simulink model "sine_test_sin_ideal"  (R2023b)
settings: Solver=FixedStepAuto  StartTime=0.0  StopTime=SimTime  FixedStep=samplingTime  RelTol=1e-3
values from neighbouring files (symbols this model uses):
  M = -max(y_norm)    [Fractional_contr.m]
  Omega = 2*pi*freq    (= 1.13097335529)    [Fractional_contr.m]
  Phi = freq*2*pi*( (27918-28129)*samplingTime )    (= -2.38635377967)    [Fractional_contr.m]
settings Model: Creator=tudor  LastModifiedBy=tudor

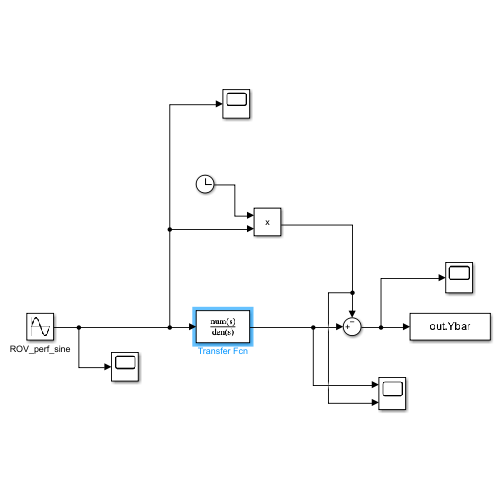
[thumbnail: Simulink's stored preview of the top-level diagram]
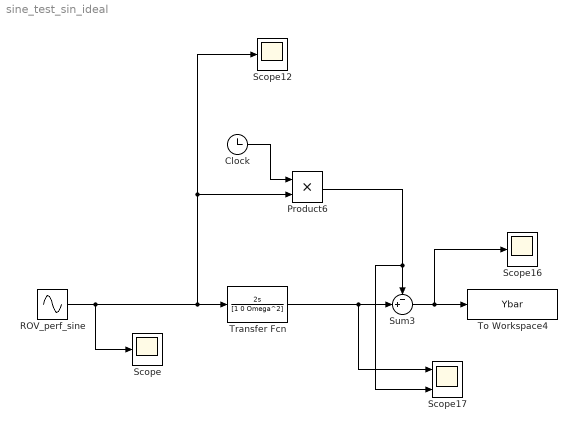
== system sine_test_sin_ideal ==
  Clock : Clock
  Product6 : Product
  ROV_perf_sine : Sin  Amplitude=M  Frequency=Omega  Phase=Phi  SampleTime=0
  Scope : Scope
  Scope12 : Scope
  Scope16 : Scope
  Scope17 : Scope  NumInputPorts=2
  Sum3 : Sum  Inputs=-+|
  To Workspace4 : ToWorkspace  VariableName=Ybar  SampleTime=-1
  Transfer Fcn : TransferFcn  Numerator=[2 0]  Denominator=[1 0 Omega^2]
  wires:
  Sum3/1 -> Scope16/1, To Workspace4/1
  Transfer Fcn/1 -> Scope17/1, Sum3/2
  Clock/1 -> Product6/1
  ROV_perf_sine/1 -> Scope/1, Scope12/1, Product6/2, Transfer Fcn/1
  Product6/1 -> Scope17/2, Sum3/1
